simulink model "Suspennsion_Model_singleWheel"  (R2020a)
settings: Solver=VariableStepAuto  StartTime=0.0  StopTime=100.0  RelTol=1e-3
values from neighbouring files (symbols this model uses):
  b = 3000    [startup_code.m]
  k1 = 16000    [startup_code.m]
  k2 = 60000    [startup_code.m]
  m1 = 2000    [startup_code.m]
  m2 = 20    [startup_code.m]
settings Model: Creator=Viraj  LastModifiedBy=Viraj

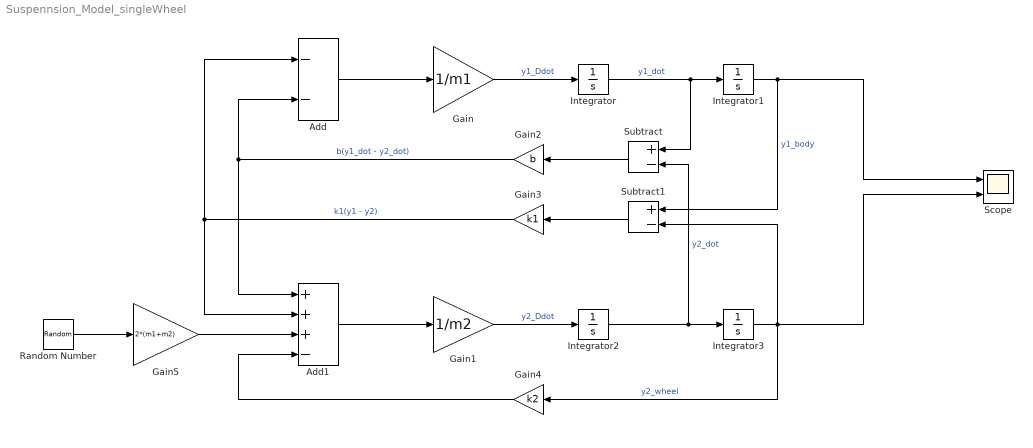
== system Suspennsion_Model_singleWheel ==
  Add : Sum  Inputs=--
  Add1 : Sum  Inputs=+++-
  Gain : Gain  Gain=1/m1
  Gain1 : Gain  Gain=1/m2
  Gain2 : Gain  Gain=b
  Gain3 : Gain  Gain=k1
  Gain4 : Gain  Gain=k2
  Gain5 : Gain  Gain=2*(m1+m2)
  Integrator{,1..3} (4 alike) : Integrator
  Random Number : RandomNumber  Seed=1  SampleTime=0.1
  Scope : Scope  NumInputPorts=2
  Subtract : Sum  Inputs=+-
  Subtract1 : Sum  Inputs=+-
  wires:
  Add/1 -> Gain/1
  Gain/1 -> Integrator/1  "y1_Ddot"
  Integrator/1 -> Subtract/1, Integrator1/1  "y1_dot"
  Gain1/1 -> Integrator2/1  "y2_Ddot"
  Add1/1 -> Gain1/1
  Integrator2/1 -> Integrator3/1, Subtract/2  "y2_dot"
  Integrator1/1 -> Subtract1/1, Scope/1  "y1_body"
  Integrator3/1 -> Gain4/1, Scope/2, Subtract1/2  "y2_wheel"
  Gain2/1 -> Add1/1, Add/2  "b(y1_dot - y2_dot)"
  Gain3/1 -> Add/1, Add1/2  "k1(y1 - y2)"
  Subtract/1 -> Gain2/1
  Subtract1/1 -> Gain3/1
  Gain4/1 -> Add1/4
  Gain5/1 -> Add1/3
  Random Number/1 -> Gain5/1
